simulink model "sim_lab_4"  (R2022b)
settings: Solver=VariableStepAuto  StartTime=0.0  StopTime=50  RelTol=1e-3
values from neighbouring files (symbols this model uses):
  a = 0.01    [run.m]
  Kr = 18    [run.m]
  Td = 1    [run.m]
  Ti = 0.55    [run.m]
settings Model: Creator=User  LastModifiedBy=radu

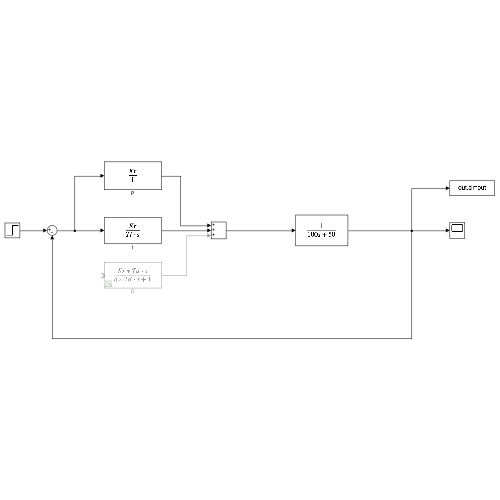
[thumbnail: Simulink's stored preview of the top-level diagram]
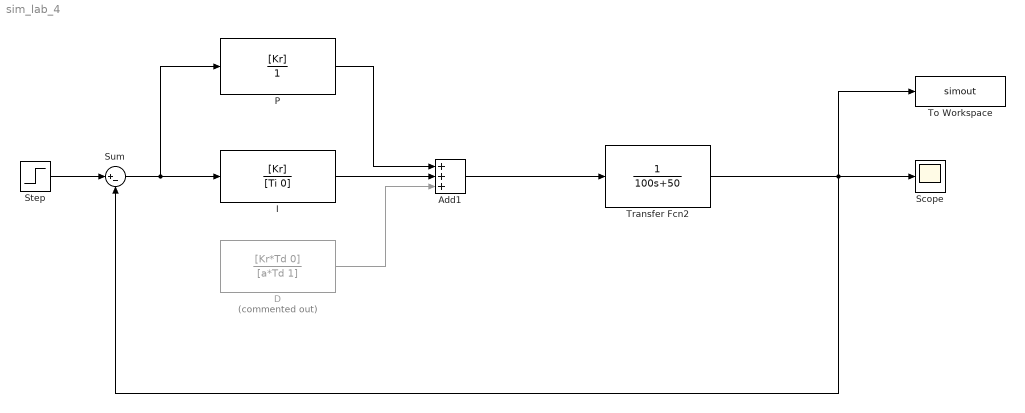
== system sim_lab_4 ==
  Add1 : Sum  Inputs=+++
  D : TransferFcn  Commented=on  Numerator=[Kr*Td 0]  Denominator=[a*Td 1]
  I : TransferFcn  Numerator=[Kr]  Denominator=[Ti 0]
  P : TransferFcn  Numerator=[Kr]  Denominator=[1]
  Scope : Scope
  Step : Step  Time=0  SampleTime=0
  Sum : Sum  Inputs=|+-
  To Workspace : ToWorkspace  VariableName=simout  SaveFormat=Timeseries  SampleTime=-1
  Transfer Fcn2 : TransferFcn  Denominator=[100 50]
  wires:
  Step/1 -> Sum/1
  Transfer Fcn2/1 -> To Workspace/1, Scope/1, Sum/2
  Add1/1 -> Transfer Fcn2/1
  Sum/1 -> I/1, P/1
  P/1 -> Add1/1
  I/1 -> Add1/2
  D/1 -> Add1/3
